simulink model "holidays13"  (R2019b)
settings: Solver=VariableStepAuto  StartTime=0.0  StopTime=20.0  RelTol=1e-3
libraries: simulink x1
settings Model: Creator=adi20  LastModifiedBy=adi20

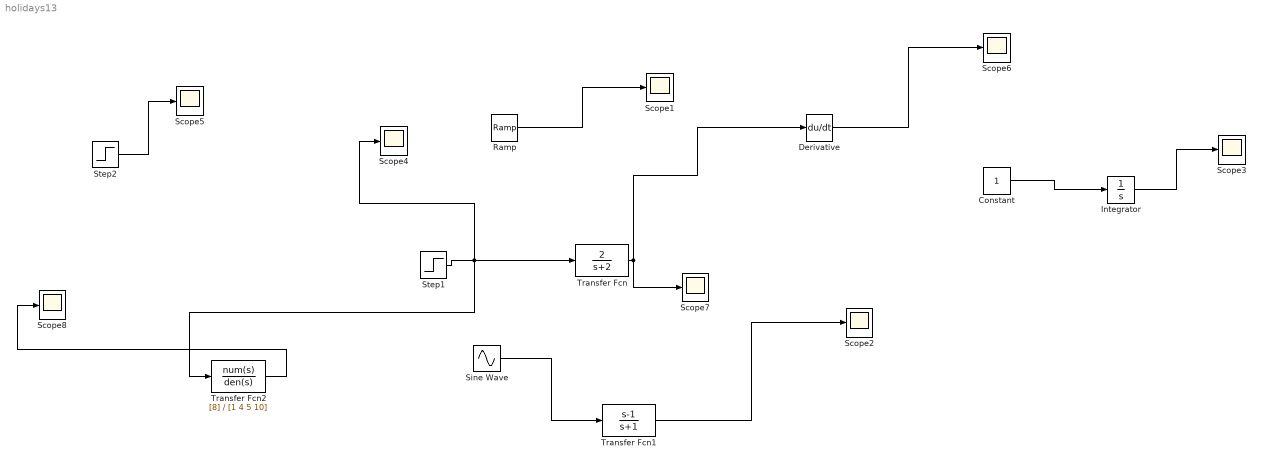
== system holidays13 ==
  Constant : Constant
  Derivative : Derivative
  Integrator : Integrator
  Ramp : simulink/Sources/Ramp  slope=1  start=0  InitialOutput=0
  Scope{1..8} (8 alike) : Scope
  Sine Wave : Sin  SampleTime=0
  Step1 : Step  Time=0  SampleTime=0
  Step2 : Step  Time=7  Before=2  After=5  SampleTime=0
  Transfer Fcn : TransferFcn  Numerator=[2]  Denominator=[1 2]
  Transfer Fcn1 : TransferFcn  Numerator=[1 -1]  Denominator=[1 1]
  Transfer Fcn2 : TransferFcn  Numerator=[8]  Denominator=[1 4 5 10]
  wires:
  Step1/1 -> Transfer Fcn2/1, Transfer Fcn/1, Scope4/1
  Transfer Fcn/1 -> Scope7/1, Derivative/1
  Ramp/1 -> Scope1/1
  Sine Wave/1 -> Transfer Fcn1/1
  Transfer Fcn1/1 -> Scope2/1
  Constant/1 -> Integrator/1
  Integrator/1 -> Scope3/1
  Step2/1 -> Scope5/1
  Derivative/1 -> Scope6/1
  Transfer Fcn2/1 -> Scope8/1
